simulink model "L3_EX2_Test"  (R2017a)
settings: Solver=VariableStepAuto  StartTime=0.0  StopTime=2  RelTol=1e-3
values from neighbouring files (symbols this model uses):
  dtot = 9.6328e-06    [L3_EX1_PI.m]
  Jtot = 2.1441e-05    [L3_EX1_PI.m]
  Kemf = 1/speedconst*60/2/pi    (= 0.0697028947848)    [L3_EX1_PI.m]
  Kt = 69.7e-3    (= 0.0697)    [L3_EX1_PI.m]
  L = 11.40e-3    (= 0.0114)    [L3_EX1_PI.m]
  R = 112    [L3_EX1_PI.m]
  Tc = 0.0016    [L3_EX1_PI.m]
libraries: cstblocks x3
settings Model: Creator=kalap  LastModifiedBy=kalap

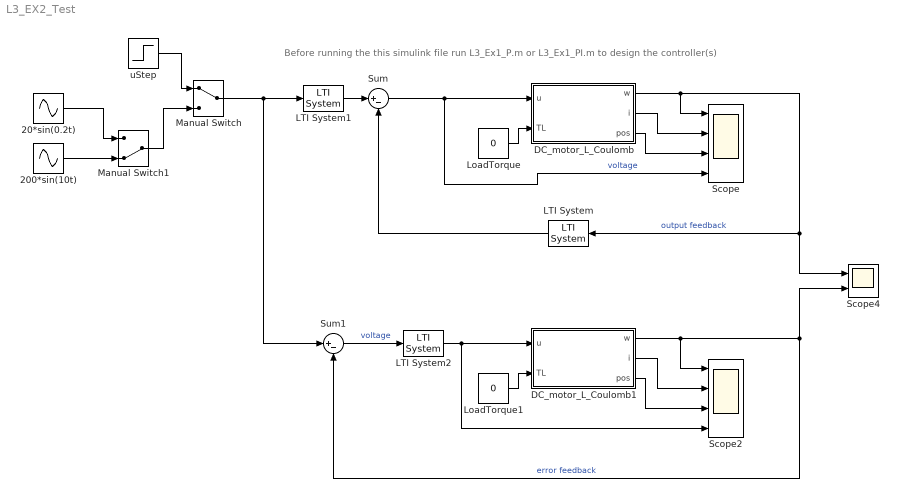
== system L3_EX2_Test ==
  note: Before running the this simulink file run L3_Ex1_P.m or L3_Ex1_PI.m to design the controller(s)
  20*sin(0.2t) : Sin  Amplitude=20  Frequency=0.2  SampleTime=0
  200*sin(10t) : Sin  Amplitude=200  Frequency=10  SampleTime=0
  DC_motor_L_Coulomb : Subsystem
  DC_motor_L_Coulomb1 : Subsystem
  LTI System : cstblocks/LTI System  sys=Hc  IC=[]
  LTI System1 : cstblocks/LTI System  sys=Hff  IC=[]
  LTI System2 : cstblocks/LTI System  sys=Hc  IC=[]
  LoadTorque : Constant  Value=0
  LoadTorque1 : Constant  Value=0
  Manual Switch : ManualSwitch
  Manual Switch1 : ManualSwitch  CurrentSetting=0
  Scope : Scope  NumInputPorts=4
  Scope2 : Scope  NumInputPorts=4
  Scope4 : Scope  NumInputPorts=2
  Sum : Sum  Inputs=|+-
  Sum1 : Sum  Inputs=|+-
  uStep : Step  After=20  SampleTime=0
  wires:
  LoadTorque/1 -> DC_motor_L_Coulomb/2(TL)
  DC_motor_L_Coulomb/2(i) -> Scope/2
  DC_motor_L_Coulomb/3(pos) -> Scope/3
  Sum/1 -> DC_motor_L_Coulomb/1(u), Scope/4  "voltage"
  LTI System/1 -> Sum/2
  LTI System1/1 -> Sum/1
  uStep/1 -> Manual Switch/1
  20*sin(0.2t)/1 -> Manual Switch1/1
  Manual Switch1/1 -> Manual Switch/2
  200*sin(10t)/1 -> Manual Switch1/2
  Sum1/1 -> LTI System2/1  "voltage"
  Manual Switch/1 -> LTI System1/1, Sum1/1
  DC_motor_L_Coulomb1/2(i) -> Scope2/2
  DC_motor_L_Coulomb1/3(pos) -> Scope2/3
  LoadTorque1/1 -> DC_motor_L_Coulomb1/2(TL)
  DC_motor_L_Coulomb1/1(w) -> Scope4/2, Sum1/2, Scope2/1  "error feedback"
  DC_motor_L_Coulomb/1(w) -> Scope/1, LTI System/1, Scope4/1  "output feedback"
  LTI System2/1 -> DC_motor_L_Coulomb1/1(u), Scope2/4

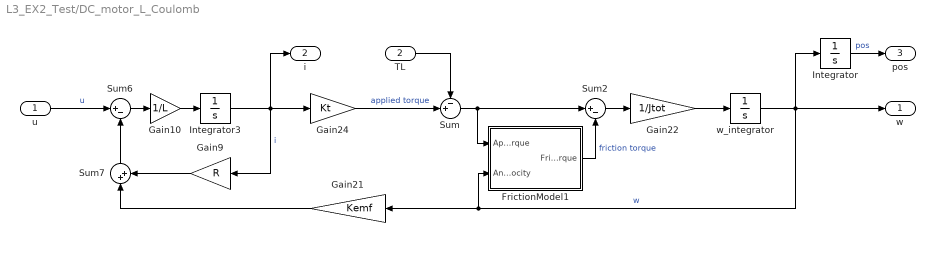
== system L3_EX2_Test/DC_motor_L_Coulomb ==
  u : Inport
  TL : Inport  Port=2
  FrictionModel1 : Subsystem
  Gain10 : Gain  Gain=1/L
  Gain21 : Gain  Gain=Kemf
  Gain22 : Gain  Gain=1/Jtot
  Gain24 : Gain  Gain=Kt
  Gain9 : Gain  Gain=R
  Integrator : Integrator
  Integrator3 : Integrator
  Sum : Sum  Inputs=-+|
  Sum2 : Sum  Inputs=|+-
  Sum6 : Sum  Inputs=|+-
  Sum7 : Sum  Inputs=|++
  w_integrator : Integrator
  w : Outport
  i : Outport  Port=2
  pos : Outport  Port=3
  wires:
  TL/1 -> Sum/1
  Gain24/1 -> Sum/2  "applied torque"
  FrictionModel1/1(Friction torque) -> Sum2/2  "friction torque"
  Sum/1 -> Sum2/1, FrictionModel1/1(Applied torque)
  Sum2/1 -> Gain22/1
  Gain22/1 -> w_integrator/1
  w_integrator/1 -> Integrator/1, w/1, FrictionModel1/2(Angular velocity), Gain21/1  "w"
  u/1 -> Sum6/1  "u"
  Gain10/1 -> Integrator3/1
  Gain9/1 -> Sum7/2
  Sum6/1 -> Gain10/1
  Gain21/1 -> Sum7/1
  Integrator3/1 -> i/1, Gain24/1, Gain9/1  "i"
  Sum7/1 -> Sum6/2
  Integrator/1 -> pos/1  "pos"

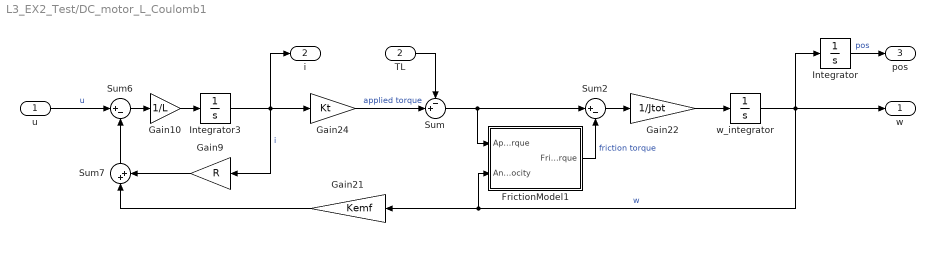
== system L3_EX2_Test/DC_motor_L_Coulomb1 ==
  u : Inport
  TL : Inport  Port=2
  FrictionModel1 : Subsystem
  Gain10 : Gain  Gain=1/L
  Gain21 : Gain  Gain=Kemf
  Gain22 : Gain  Gain=1/Jtot
  Gain24 : Gain  Gain=Kt
  Gain9 : Gain  Gain=R
  Integrator : Integrator
  Integrator3 : Integrator
  Sum : Sum  Inputs=-+|
  Sum2 : Sum  Inputs=|+-
  Sum6 : Sum  Inputs=|+-
  Sum7 : Sum  Inputs=|++
  w_integrator : Integrator
  w : Outport
  i : Outport  Port=2
  pos : Outport  Port=3
  wires:
  TL/1 -> Sum/1
  Gain24/1 -> Sum/2  "applied torque"
  FrictionModel1/1(Friction torque) -> Sum2/2  "friction torque"
  Sum/1 -> Sum2/1, FrictionModel1/1(Applied torque)
  Sum2/1 -> Gain22/1
  Gain22/1 -> w_integrator/1
  w_integrator/1 -> Integrator/1, w/1, FrictionModel1/2(Angular velocity), Gain21/1  "w"
  u/1 -> Sum6/1  "u"
  Gain10/1 -> Integrator3/1
  Gain9/1 -> Sum7/2
  Sum6/1 -> Gain10/1
  Gain21/1 -> Sum7/1
  Integrator3/1 -> i/1, Gain24/1, Gain9/1  "i"
  Sum7/1 -> Sum6/2
  Integrator/1 -> pos/1  "pos"

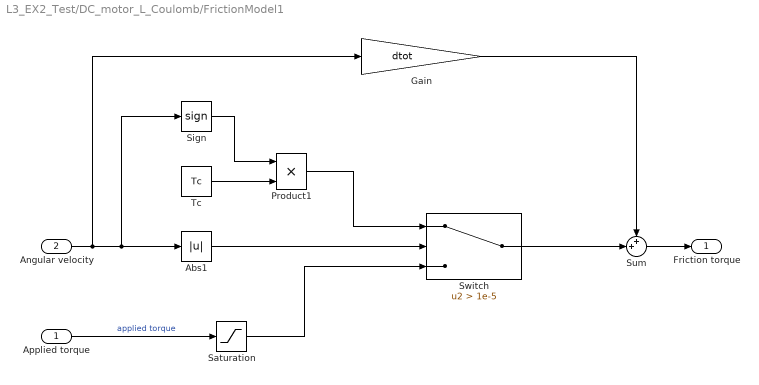
== system L3_EX2_Test/DC_motor_L_Coulomb/FrictionModel1 ==
  Applied torque : Inport
  Angular velocity : Inport  Port=2
  Abs1 : Abs
  Gain : Gain  Gain=dtot
  Product1 : Product
  Saturation : Saturate  UpperLimit=Tc  LowerLimit=-Tc
  Sign : Signum
  Sum : Sum  Inputs=++|
  Switch : Switch  Criteria=u2 > Threshold  Threshold=1e-5
  Tc : Constant  Value=Tc
  Friction torque : Outport
  wires:
  Angular velocity/1 -> Gain/1, Sign/1, Abs1/1
  Sign/1 -> Product1/1
  Applied torque/1 -> Saturation/1  "applied torque"
  Abs1/1 -> Switch/2
  Tc/1 -> Product1/2
  Product1/1 -> Switch/1
  Switch/1 -> Sum/2
  Saturation/1 -> Switch/3
  Sum/1 -> Friction torque/1
  Gain/1 -> Sum/1

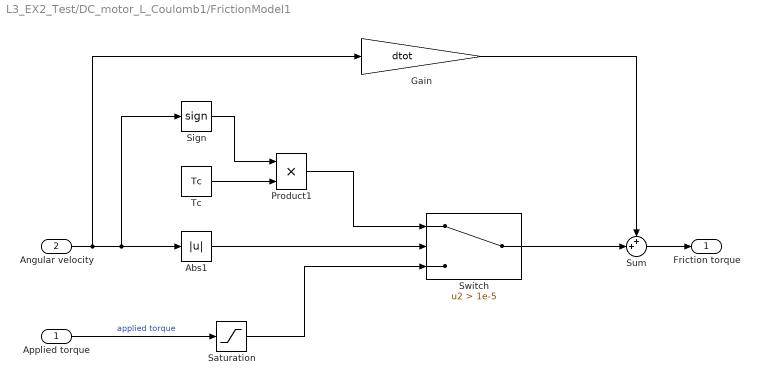
== system L3_EX2_Test/DC_motor_L_Coulomb1/FrictionModel1 ==
  Applied torque : Inport
  Angular velocity : Inport  Port=2
  Abs1 : Abs
  Gain : Gain  Gain=dtot
  Product1 : Product
  Saturation : Saturate  UpperLimit=Tc  LowerLimit=-Tc
  Sign : Signum
  Sum : Sum  Inputs=++|
  Switch : Switch  Criteria=u2 > Threshold  Threshold=1e-5
  Tc : Constant  Value=Tc
  Friction torque : Outport
  wires:
  Angular velocity/1 -> Gain/1, Sign/1, Abs1/1
  Sign/1 -> Product1/1
  Applied torque/1 -> Saturation/1  "applied torque"
  Abs1/1 -> Switch/2
  Tc/1 -> Product1/2
  Product1/1 -> Switch/1
  Switch/1 -> Sum/2
  Saturation/1 -> Switch/3
  Sum/1 -> Friction torque/1
  Gain/1 -> Sum/1
